simulink model "SUB_CanDm1"  (R2018b)
settings: Solver=VariableStepDiscrete  StartTime=0.0  StopTime=10  RelTol=1e-3
PreLoadFcn:
  | if(exist('MBDS_ModelCallback', 'file'))
  |    MBDS_ModelCallback('PreLoad');
  | end
PostLoadFcn:
  | if(exist('MBDS_ModelCallback', 'file'))
  |    MBDS_ModelCallback('PostLoad');
  | end
InitFcn:
  | if(exist('MBDS_ModelCallback', 'file'))
  |    MBDS_ModelCallback('Init');
  | end
StartFcn:
  | if(exist('MBDS_ModelCallback', 'file'))
  |    MBDS_ModelCallback('Start');
  | end
StopFcn:
  | if(exist('MBDS_ModelCallback', 'file'))
  |    MBDS_ModelCallback('Stop');
  | end
undefined symbols (not defined in the file): sigbuilder_block
libraries: KIBES_Signal x47, simulink x1
(part 1 of 2)
PreSaveFcn:
  | if(exist('MBDS_ModelCallback', 'file'))
  |    MBDS_ModelCallback('PreSave');
  | end
CloseFcn:
  | if(exist('MBDS_ModelCallback', 'file'))
  |    MBDS_ModelCallback('Close');
  | end
Description:
  | Design model of an MBDS Subsystem
settings Model: IsTargetCode=false  MBDS_Version=08.20  Creator=Marcio Kopke (uid96494)  LastModifiedBy=uid96494
settings ConfigSet: Description=MBDS configuration set optimized for simulation of model designs for automotive embedded systems.
settings SolverCC: MinimalZcImpactIntegration=on
settings DataIOCC: MaxDataPoints=100  SaveFormat=StructureWithTime  SaveOutput=off  DSMLogging=off  VisualizeSimOutput=off  SaveTime=off  SignalLoggingName=LogSignals
settings OptimizationCC: UseDivisionForNetSlopeComputation=UseDivisionForReciprocalsOfIntegersOnly  UseFloatMulNetSlope=on  DefaultUnderspecifiedDataType=single  OptimizeBlockIOStorage=off  BufferReuse=off  GlobalBufferReuse=off  StrengthReduction=on  ExpressionFolding=off  ExpressionDepthLimit=2147483647  LocalBlockOutputs=off  EfficientFloat2IntCast=on  LifeSpan=inf  BufferReusableBoundary=off  OptimizeBlockOrder=speed  OptimizeDataStoreBuffers=off  BusAssignmentInplaceUpdate=off  LabelGuidedReuse=on
settings DebuggingCC: SignalInfNanChecking=error  AlgebraicLoopMsg=error  ArtificialAlgebraicLoopMsg=error  UnderspecifiedInitializationDetection=Classic  CheckExecutionContextPreStartOutputMsg=on  CheckExecutionContextRuntimeOutputMsg=on  BlockPriorityViolationMsg=error  MinStepSizeMsg=error  TimeAdjustmentMsg=warning  SolverPrmCheckMsg=error  InheritedTsInSrcMsg=none  SingleTaskRateTransMsg=error  TasksWithSamePriorityMsg=error  SigSpecEnsureSampleTimeMsg=error  CheckMatrixSingularityMsg=error  ParameterUnderflowMsg=error  ParameterTunabilityLossMsg=error  FixptConstUnderflowMsg=warning  FixptConstOverflowMsg=warning  FixptConstPrecisionLossMsg=warning  VectorMatrixConversionMsg=error  SignalLabelMismatchMsg=warning  SFcnCompatibilityMsg=error  FrameProcessingCompatibilityMsg=warning  UniqueDataStoreMsg=error  BusObjectLabelMismatch=error  RootOutportRequireBusObject=error  AllowSymbolicDim=off  ModelReferenceIOMsg=error  ModelReferenceIOMismatchMessage=error  UnknownTsInhSupMsg=error  ModelReferenceDataLoggingMessage=error  StateNameClashWarn=warning  SimStateOlderReleaseMsg=warning  StrictBusMsg=ErrorOnBusTreatedAsVector  NonBusSignalsTreatedAsBus=error  SFInvalidInputDataAccessInChartInitDiag=error  SFTransitionOutsideNaturalParentDiag=error  SFUnreachableExecutionPathDiag=error  SFUndirectedBroadcastEventsDiag=error  SFTransitionActionBeforeConditionDiag=error  SFTemporalDelaySmallerThanSampleTimeDiag=error  SFExecutionAtInitializationDiag=none
settings HardwareCC: ProdBitPerPointer=32  ProdBitPerSizeT=32  ProdBitPerPtrDiffT=32  ProdLargestAtomicInteger=Long  ProdEndianess=BigEndian  ProdWordSize=32  ProdLongLongMode=on  ProdHWDeviceType=Custom Processor  TargetHWDeviceType=32-bit Generic
settings ModelReferenceCC: PropagateSignalLabelsOutOfModel=off
settings SFSimCC: SimUseLocalCustomCode=off  SimGenImportedTypeDefs=on  CompileTimeRecursionLimit=0  EnableRuntimeRecursion=off  MATLABDynamicMemAlloc=off  DefaultCustomCodeFunctionArrayLayout=Column-major
settings RTWCC: SystemTargetFile=MBDS.tlc  GenCodeOnly=on  TemplateMakefile=MBDS.tmf  Description=MBDS Target  GenerateReport=on  RTWUseLocalCustomCode=off  IncludeHyperlinkInReport=on  LaunchReport=on  GenerateTraceReport=on  GenerateTraceReportSl=on  GenerateTraceReportSf=on  GenerateTraceReportEml=on  GenerateCodeMetricsReport=on  RTWCompilerOptimization=on
settings CodeAppCC: ForceParamTrailComments=on  IgnoreCustomStorageClasses=off  OperatorAnnotations=on  SimulinkDataObjDesc=on  SFDataObjDesc=on  MangleLength=2  CustomSymbolStrType=$N$R$M  CustomSymbolStrFcn=$R$M  CustomSymbolStrUtil=$n$C  InsertBlockDesc=on  StateflowObjectComments=on  MATLABSourceComments=on  ReqsInCode=on  UseSimReservedNames=on
settings STFCustomTargetCC: UtilityFuncGeneration=Shared location  MultiwordLength=256  DynamicStringBufferSize=2  InferredTypesCompatibility=on  ModelReferenceCompliant=off  IncludeMdlTerminateFcn=off  CombineOutputUpdateFcns=on  CombineSignalStateStructs=on  SuppressErrorStatus=on  ERTCustomFileBanners=on  SupportComplex=off  SupportContinuousTime=off  SupportNonInlinedSFcns=off  RemoveDisableFunc=on  RemoveResetFunc=on  ParenthesesLevel=Maximum  CastingMode=Standards  MATLABClassNameForMDSCustomization=Simulink.SoftwareTarget.ERTCustomization  GenerateSharedConstants=off  SystemTargetFile=MBDS.tlc
settings ERTTargetCC: UtilityFuncGeneration=Shared location  DynamicStringBufferSize=2  InferredTypesCompatibility=on  ModelReferenceCompliant=off  ParMdlRefBuildCompliant=off  CompOptLevelCompliant=off  ConcurrentExecutionCompliant=off  IncludeMdlTerminateFcn=off  CombineSignalStateStructs=on  SuppressErrorStatus=on  SupportComplex=off  RemoveDisableFunc=on  ParenthesesLevel=Maximum  CastingMode=Standards  ModelStepFunctionPrototypeControlCompliant=off  CPPClassGenCompliant=off  UseToolchainInfoCompliant=off  GenerateSharedConstants=off  ERTCustomFileTemplate=example_file_process.tlc  EnableDataOwnership=on  PreserveExpressionOrder=on  PreserveIfCondition=on  SuppressUnreachableDefaultCases=off  EnableSignedLeftShifts=off  EnableSignedRightShifts=off  IndentStyle=Allman  NewlineStyle=CR+LF
settings ConfigComp: CovScope=ReferencedModels  CovIncludeTopModel=off  CovPath=SUB_CanDm1/Model/SUB_CanDm1_  CovSaveName=covData  CovMetricSettings=dsw  CovFilter=MBDS_CoverageFilter  CovHTMLOptions=-sRT=1 -sVT=0 -aTS=1 -bRG=1 -bTC=1 -hTR=1 -nFC=0 -nFD=0 -scm=1 -bcm=1 -xEv=0 -xEM=1  CovHtmlReporting=on  CovSaveOutputData=off  CovDataFileName=covData  CovShowResultsExplorer=off  CovExternalEMLEnable=off  CovSFcnEnable=off

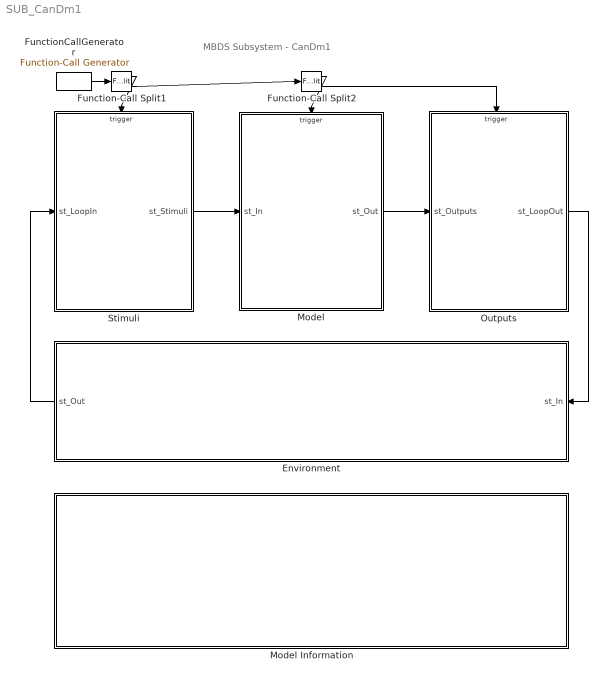
== system SUB_CanDm1 ==
  note: MBDS Subsystem - CanDm1
  Environment : Subsystem  Description=Environment subsystem for a MBDS model.
  Function-Call Split1 : FunctionCallSplit  InitFcn=|  NumOutputPorts=2
      | try
      |    MBDS_BlockCallback('Update', gcb);
      | end
      | try
      |    MBDS_BlockCallback('Update', gcb);
      | end
  Function-Call Split2 : FunctionCallSplit  InitFcn=|  NumOutputPorts=2
      | try
      |    MBDS_BlockCallback('Update', gcb);
      | end
      | try
      |    MBDS_BlockCallback('Update', gcb);
      | end
  FunctionCallGenerator : simulink/Ports & Subsystems/Function-Call Generator  sample_time=0.01  numberOfIterations=1
      settings: AttributesFormatString=Ts = %<sample_time>
  Model : Subsystem  Description=Model subsystem for a MBDS model. Here, the input signals to the model functionality are resolved from the Stimuli bus and the output signals of the model functionality are summarized into the Results bus.
  Model Information : Subsystem  InitFcn=|  mask(ModelInformation){MBDS_LibraryBlock=on, Company=-, Department=-, Responsible=-, Status=In Work, Complete=on, Check=on, Test=on, Optimize=on, Documentation=on, FcnErrors=off, GenericToDo=off, DocumentState=Draft, GenericToDoName=Enter a user specific ToDo text, MBDS_BlockVersion=07.00}
      | if(exist('MBDS_BlockCallback', 'file'))
      |    MBDS_BlockCallback('Update', gcb);
      | end
      mask prompts: MBDS_LibraryBlock "MBDS Library Block"; Complete "Complete Implementation"; Check "Check Modelling Guidelines"; Test "Test Functionality"; Optimize "Optimize Implementation"; Documentation "Create Documentation"; FcnErrors "Remove Functional Errors"; GenericToDo "Enter a user specific ToDo text"; DocumentState "Document State:"; GenericToDoName "Generic ToDo Name:"; MBDS_BlockVersion "Block version:"
      mask help: This block displays model information and ToDo's on it's block mask. Via the block parameter mask further model information and configuration options can be accessed.
      mask init:
      | if(exist('MBDS_BlockCallback', 'file'))
      |    MBDS_BlockCallback('Copy', gcb);    
      | end
      mask Help: eval(['open([workdir(''library_dir:''),''\Blockset\help\'',get_param(gcb,''MaskType''),''.html''])'])
      mask TypeOptions Status: In Work | Done
      mask TypeOptions DocumentState: Draft | Final | Released
      mask Callback GenericToDoName:
      | MaskPrompts = get_param(gcb, 'MaskPrompts');
      | MaskPrompts{12} = get_param(gcb, 'GenericToDoName');
      | if(length(MaskPrompts{12}) > 75)
      |    MaskPrompts{12} = MaskPrompts{12}(1:75);
      |    set_param(gcb, 'GenericToDoName', MaskPrompts{12});
      | end
      | set_param(gcb, 'MaskPrompts', MaskPrompts);
      | clear MaskPrompts;
      mask DialogControl ParameterTabVar0 Prompt: Info
      mask DialogControl ParameterTabVar01 Prompt: ToDo's
      mask DialogControl ParameterTabVar012 Prompt: Options
      mask DialogControl ParameterTabVar0123 Prompt: Version
      mask Display:
      | % Get ToDo's
      | IsComplete       = strcmpi(Complete, 'on');
      | IsOptimize       = strcmpi(Optimize, 'on');
      | IsCheck          = strcmpi(Check, 'on');
      | IsDocumentation  = strcmpi(Documentation, 'on');
      | IsTest           = strcmpi(Test, 'on');
      | IsFcnErrors      = strcmpi(FcnErrors, 'on');
      | IsGenericToDo    = strcmpi(GenericToDo, 'on');
      | 
      | % Determine status
      | if(IsFcnErrors || IsTest || IsComplete || IsDocumentation || IsCheck || IsOptimize || IsGenericToDo)
      |    Status = 'In Work';
      | else
      |    Status = 'Done';
      | end
      | 
      | % Update status parameter
      | if(~strcmpi(get_param(gcb, 'Status'), Status))
      |    set_param(gcb, 'Status', Status);
      | end
      | 
      | % Determine severity
      | if(IsFcnErrors)
      |    % Severity: Critical
      |    BoxColorFile = 'Box_Red.tif';
      |    IconFile     = 'State_Red.jpg';
      | elseif (IsTest || IsComplete || IsGenericToDo)
      |    % Severity: Major
      |    BoxColorFile = 'Box_Orange.tif';
      |    IconFile     = 'State_Orange.jpg';
      | elseif (IsDocumentation || IsCheck || IsOptimize)
      |    % Severity: Minor
      |    BoxColorFile = 'Box_Grey.tif';
      |    IconFile     = 'State_Grey.jpg';
      | else
      |    % Severity: None
      |    BoxColorFile = 'Box_Green.tif';
      |    IconFile     = 'State_Green.jpg';
      | end
      | 
      | % Display Model Information
      | InfoStr1 = sprintf('%s', get_param(bdroot, 'Name'));
      | InfoStr2 = sprintf('Model Version:  %s', get_param(bdroot, 'ModelVersion'));
      | InfoStr3 = sprintf('Company:  %s', Company);
      | InfoStr4 = sprintf('Department:  %s', Department);
      | InfoStr5 = sprintf('Responsible:  %s', Responsible);
      | InfoStr6 = sprintf('Last Modified by:  %s at %s', get_param(bdroot, 'LastModifiedBy'), get_param(bdroot, 'LastModifiedDate'));
      | %Y is to do!!!!
      | text(0.5, 0.69, sprintf('%s\n%s\n%s\n%s\n%s\n%s\n%s', InfoStr1, InfoStr2, InfoStr3, InfoStr4, InfoStr5, InfoStr6), 'horizontalAlignment', 'center');
      | clear InfoStr1 InfoStr2 InfoStr3 InfoStr4 InfoStr5 InfoStr6;
      | 
      | % Display Status
      | if(exist(BoxColorFile, 'file'))
      |    image(imread(BoxColorFile,'tif'), [0,0,1,0.45]);
      | end
      | if(exist(IconFile, 'file'))
      |    image(imread(IconFile,'jpg'), [0.025,0.09,0.08,0.26]);
      |    image(imread(IconFile,'jpg'), [0.9,0.09,0.08,0.26]);
      | end
      | plot([-0.01 1.01], [0.45 0.45])
      | text(0.5, 0.38, sprintf('Status: %s', upper(Status)), 'horizontalAlignment', 'center');
      | 
      | % Display ToDo's
      | if(IsComplete)
      |    text(0.15, 0.31, '- Complete Implementation');
      | end
      | if(IsOptimize)
      |    text(0.6, 0.31, '- Optimize Implementation');
      | end
      | 
      | if(IsCheck)
      |    text(0.15, 0.23, '- Check Modeling Guidelines');
      | end
      | if(IsDocumentation)
      |    text(0.6, 0.23, '- Create Documentation');
      | end
      | 
      | if(IsTest)
      |    text(0.15, 0.14, '- Test Functionality');
      | end
      | if(IsFcnErrors)
      |    text(0.6, 0.14, '- Remove Functional Errors');
      | end
      | 
      | if(IsGenericToDo)
      |    text(0.15, 0.06, ['- ', GenericToDoName]);
      | end
  Outputs : Subsystem  Description=Result subsystem for a MBDS model. Here, output signals from the model functionality can be displayed using a scope or display. Additionally, the output signals can be postprocessed before they will passed to the feedback loop.
  Stimuli : Subsystem  Description=Stimuli subsystem for a MBDS model. Here, input signals for testing the model functionality can be defined using the signal builder or calculated applying arbitrary basic-blocks. Additionally, feedback signals can be preprocessed at this stage.
  wires:
  Model/1(st_Out) -> Outputs/1(st_Outputs)
  Stimuli/1(st_Stimuli) -> Model/1(st_In)
  Outputs/1(st_LoopOut) -> Environment/1(st_In)
  Environment/1(st_Out) -> Stimuli/1(st_LoopIn)
  FunctionCallGenerator/1 -> Function-Call Split1/1
  Function-Call Split1/2 -> Function-Call Split2/1
  Function-Call Split1/1 -> Stimuli/Trigger
  Function-Call Split2/1 -> Model/Trigger
  Function-Call Split2/2 -> Outputs/Trigger

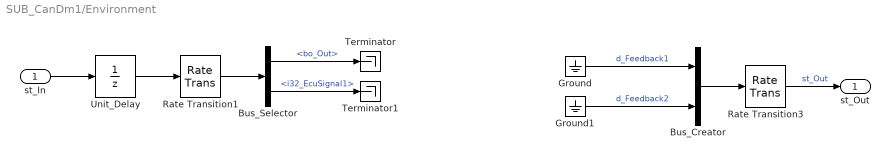
== system SUB_CanDm1/Environment ==
  st_In : Inport
  Bus_Creator : BusCreator  InitFcn=|  Inputs=2
      | try
      |    MBDS_BlockCallback('Update', gcb);
      | end
      | try
      |    MBDS_BlockCallback('Update', gcb);
      | end
  Bus_Selector : BusSelector  InitFcn=|  OutputSignals=st_Outputs.bo_Out,i32_EcuSignal1
      | try
      |    MBDS_BlockCallback('Update', gcb);
      | end
      | try
      |    MBDS_BlockCallback('Update', gcb);
      | end
  Ground : Ground  InitFcn=|
      | try
      |    MBDS_BlockCallback('Update', gcb);
      | end
  Ground1 : Ground  InitFcn=|
      | try
      |    MBDS_BlockCallback('Update', gcb);
      | end
  Rate Transition1 : RateTransition  InitFcn=|  OutPortSampleTimeOpt=Inherit
      | try
      |    MBDS_BlockCallback('Update', gcb);
      | end
  Rate Transition3 : RateTransition  InitFcn=|  OutPortSampleTimeOpt=Inherit
      | try
      |    MBDS_BlockCallback('Update', gcb);
      | end
  Terminator : Terminator
      settings: MoveFcn=UpdateBlockSize(gcb);
      settings: InitFcn=|
      | try
      |    MBDS_BlockCallback('Update', gcb);
      | end
  Terminator1 : Terminator
      settings: MoveFcn=UpdateBlockSize(gcb);
      settings: InitFcn=|
      | try
      |    MBDS_BlockCallback('Update', gcb);
      | end
  Unit_Delay : UnitDelay  InitFcn=|  SampleTime=-1
      | try
      |    MBDS_BlockCallback('Update', gcb);
      | end
      | try                                  
      |    MBDS_BlockCallback('Update', gcb);
      | end
      settings: AttributesFormatString=Init = %<X0>
  st_Out : Outport
  wires:
  Bus_Creator/1 -> Rate Transition3/1
  st_In/1 -> Unit_Delay/1
  Ground/1 -> Bus_Creator/1  "d_Feedback1"
  Ground1/1 -> Bus_Creator/2  "d_Feedback2"
  Unit_Delay/1 -> Rate Transition1/1
  Rate Transition3/1 -> st_Out/1  "st_Out"
  Rate Transition1/1 -> Bus_Selector/1
  Bus_Selector/1 -> Terminator/1  "<bo_Out>"
  Bus_Selector/2 -> Terminator1/1  "<i32_EcuSignal1>"

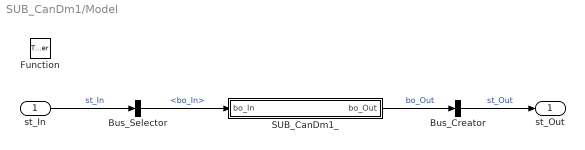
== system SUB_CanDm1/Model ==
  st_In : Inport
      settings: LatchInputForFeedbackSignals=on
  Function : TriggerPort  InitFcn=|  TriggerType=function-call  VariantControl=(inherit)
      | try
      |    MBDS_BlockCallback('Update', gcb);
      | end
  Bus_Creator : BusCreator  InitFcn=|  Inputs=1
      | try
      |    MBDS_BlockCallback('Update', gcb);
      | end
      | try
      |    MBDS_BlockCallback('Update', gcb);
      | end
  Bus_Selector : BusSelector  InitFcn=|  OutputSignals=bo_In
      | try
      |    MBDS_BlockCallback('Update', gcb);
      | end
      | try
      |    MBDS_BlockCallback('Update', gcb);
      | end
  SUB_CanDm1_ : Subsystem  Tag=Functionality  Description=Check DM1 Rx/Tx
      settings: AttributesFormatString=Functionality
  st_Out : Outport
  wires:
  st_In/1 -> Bus_Selector/1  "st_In"
  Bus_Creator/1 -> st_Out/1  "st_Out"
  Bus_Selector/1 -> SUB_CanDm1_/1(bo_In)  "<bo_In>"
  SUB_CanDm1_/1(bo_Out) -> Bus_Creator/1  "bo_Out"

== system SUB_CanDm1/Model Information ==
  note: Double Click the Model Information block to open the block parameter mask

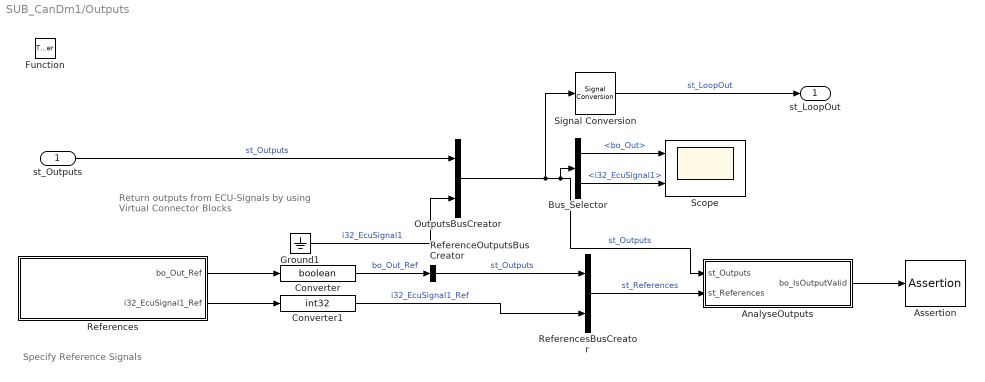
== system SUB_CanDm1/Outputs ==
  note: Specify Reference Signals
  note: Return outputs from ECU-Signals
      | by using Virtual Connector Blocks
  st_Outputs : Inport
      settings: LatchInputForFeedbackSignals=on
  Function : TriggerPort  InitFcn=|  TriggerType=function-call  VariantControl=(inherit)
      | try
      |    MBDS_BlockCallback('Update', gcb);
      | end
  AnalyseOutputs : Subsystem
  Assertion : Assertion  Enabled=off
  Bus_Selector : BusSelector  InitFcn=|  OutputSignals=st_Outputs.bo_Out,i32_EcuSignal1
      | try
      |    MBDS_BlockCallback('Update', gcb);
      | end
      | try
      |    MBDS_BlockCallback('Update', gcb);
      | end
  Converter : DataTypeConversion  InitFcn=|  OutDataTypeStr=boolean  SaturateOnIntegerOverflow=on
      | try
      |    MBDS_BlockCallback('Update', gcb);
      | end
      settings: AttributesFormatString=Saturate: %<SaturateOnIntegerOverflow>
  Converter1 : DataTypeConversion  InitFcn=|  OutDataTypeStr=int32  SaturateOnIntegerOverflow=on
      | try
      |    MBDS_BlockCallback('Update', gcb);
      | end
      settings: AttributesFormatString=Saturate: %<SaturateOnIntegerOverflow>
  Ground1 : Ground  InitFcn=|
      | try
      |    MBDS_BlockCallback('Update', gcb);
      | end
      | try
      |    MBDS_BlockCallback('Update', gcb);
      | end
  OutputsBusCreator : BusCreator  InitFcn=|  Inputs=2
      | try
      |    MBDS_BlockCallback('Update', gcb);
      | end
      | try
      |    MBDS_BlockCallback('Update', gcb);
      | end
  ReferenceOutputsBusCreator : BusCreator  InitFcn=|  Inputs=1
      | try
      |    MBDS_BlockCallback('Update', gcb);
      | end
      | try
      |    MBDS_BlockCallback('Update', gcb);
      | end
  References : Subsystem  Tag=STV Subsys  LoadFcn=sigbuilder_block('load');  StartFcn=sigbuilder_block('start');  StopFcn=sigbuilder_block('stop');  ClipboardFcn=sigbuilder_block('clipboard');  mask(Sigbuilder block){tuvar=[0:10]}
      mask init:
      | if ~strcmp(get_param(bdroot(gcb),'SimulationStatus'),'stopped'),tuvar = sigbuilder_block('maskInit'); end
      settings: CopyFcn=sigbuilder_block('copy');  DeleteFcn=sigbuilder_block('delete');  ModelCloseFcn=sigbuilder_block('modelClose');  PreSaveFcn=sigbuilder_block('preSave');  PauseFcn=sigbuilder_block('pause');  ContinueFcn=sigbuilder_block('continue');  NameChangeFcn=sigbuilder_block('namechange');  OpenFcn=sigbuilder_block('open',[50 50 520 400 ]);  CloseFcn=sigbuilder_block('close');
      mask Display: plot(0, 0, 100, 100,[2, 2, 32, 32, 2], [68, 8, 8, 68, 68],[32, 2], [38, 38], [32, 19, 2],[53, 60, 44], [32, 17, 17, 2],[16, 16, 31, 31]);txt = getActiveGroup(gcbh);text(2, 100, txt,'verticalAlignment', 'top');
  ReferencesBusCreator : BusCreator  InitFcn=|  Inputs=2
      | try
      |    MBDS_BlockCallback('Update', gcb);
      | end
      | try
      |    MBDS_BlockCallback('Update', gcb);
      | end
  Scope : Scope  NumInputPorts=2
  Signal Conversion : SignalConversion  InitFcn=|  OverrideOpt=off
      | try
      |    MBDS_BlockCallback('Update', gcb);
      | end
  st_LoopOut : Outport
  wires:
  AnalyseOutputs/1(bo_IsOutputValid) -> Assertion/1
  ReferencesBusCreator/1 -> AnalyseOutputs/2(st_References)  "st_References"
  st_Outputs/1 -> OutputsBusCreator/1  "st_Outputs"
  Ground1/1 -> OutputsBusCreator/2  "i32_EcuSignal1"
  OutputsBusCreator/1 -> AnalyseOutputs/1(st_Outputs), Bus_Selector/1, Signal Conversion/1  "st_Outputs"
  Signal Conversion/1 -> st_LoopOut/1  "st_LoopOut"
  Bus_Selector/1 -> Scope/1  "<bo_Out>"
  Bus_Selector/2 -> Scope/2  "<i32_EcuSignal1>"
  ReferenceOutputsBusCreator/1 -> ReferencesBusCreator/1  "st_Outputs"
  Converter/1 -> ReferenceOutputsBusCreator/1  "bo_Out_Ref"
  References/1(bo_Out_Ref) -> Converter/1
  References/2(i32_EcuSignal1_Ref) -> Converter1/1
  Converter1/1 -> ReferencesBusCreator/2  "i32_EcuSignal1_Ref"

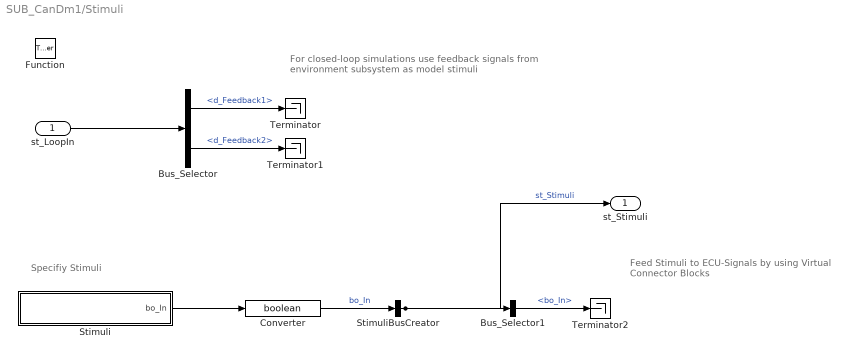
== system SUB_CanDm1/Stimuli ==
  note: Specifiy Stimuli
  note: For closed-loop simulations use feedback signals
      | from environment subsystem as model stimuli
  note: Feed Stimuli to ECU-Signals
      | by using Virtual Connector Blocks
  st_LoopIn : Inport
      settings: LatchInputForFeedbackSignals=on
  Function : TriggerPort  InitFcn=|  TriggerType=function-call  VariantControl=(inherit)
      | try
      |    MBDS_BlockCallback('Update', gcb);
      | end
  Bus_Selector : BusSelector  InitFcn=|  OutputSignals=d_Feedback1,d_Feedback2
      | try
      |    MBDS_BlockCallback('Update', gcb);
      | end
      | try
      |    MBDS_BlockCallback('Update', gcb);
      | end
  Bus_Selector1 : BusSelector  InitFcn=|  OutputSignals=bo_In
      | try
      |    MBDS_BlockCallback('Update', gcb);
      | end
      | try
      |    MBDS_BlockCallback('Update', gcb);
      | end
  Converter : DataTypeConversion  InitFcn=|  OutDataTypeStr=boolean  SaturateOnIntegerOverflow=on
      | try
      |    MBDS_BlockCallback('Update', gcb);
      | end
      settings: AttributesFormatString=Saturate: %<SaturateOnIntegerOverflow>
  Stimuli : Subsystem  Tag=STV Subsys  LoadFcn=sigbuilder_block('load');  StartFcn=sigbuilder_block('start');  StopFcn=sigbuilder_block('stop');  ClipboardFcn=sigbuilder_block('clipboard');  mask(Sigbuilder block){tuvar=[0:10]}
      mask init:
      | if ~strcmp(get_param(bdroot(gcb),'SimulationStatus'),'stopped'),tuvar = sigbuilder_block('maskInit'); end
      settings: CopyFcn=sigbuilder_block('copy');  DeleteFcn=sigbuilder_block('delete');  ModelCloseFcn=sigbuilder_block('modelClose');  PreSaveFcn=sigbuilder_block('preSave');  PauseFcn=sigbuilder_block('pause');  ContinueFcn=sigbuilder_block('continue');  NameChangeFcn=sigbuilder_block('namechange');  OpenFcn=sigbuilder_block('open',[50 50 520 400 ]);  CloseFcn=sigbuilder_block('close');
      mask Display: plot(0, 0, 100, 100,[2, 2, 32, 32, 2], [68, 8, 8, 68, 68],[32, 2], [38, 38], [32, 19, 2],[53, 60, 44], [32, 17, 17, 2],[16, 16, 31, 31]);txt = getActiveGroup(gcbh);text(2, 100, txt,'verticalAlignment', 'top');
  StimuliBusCreator : BusCreator  InitFcn=|  Inputs=1
      | try
      |    MBDS_BlockCallback('Update', gcb);
      | end
      | try
      |    MBDS_BlockCallback('Update', gcb);
      | end
  Terminator : Terminator
      settings: InitFcn=|
      | try
      |    MBDS_BlockCallback('Update', gcb);
      | end
      | try
      |    MBDS_BlockCallback('Update', gcb);
      | end
  Terminator1 : Terminator
      settings: InitFcn=|
      | try
      |    MBDS_BlockCallback('Update', gcb);
      | end
      | try
      |    MBDS_BlockCallback('Update', gcb);
      | end
  Terminator2 : Terminator
      settings: MoveFcn=UpdateBlockSize(gcb);
      settings: InitFcn=|
      | try
      |    MBDS_BlockCallback('Update', gcb);
      | end
  st_Stimuli : Outport
  wires:
  Bus_Selector/1 -> Terminator/1  "<d_Feedback1>"
  Bus_Selector/2 -> Terminator1/1  "<d_Feedback2>"
  st_LoopIn/1 -> Bus_Selector/1
  Bus_Selector1/1 -> Terminator2/1  "<bo_In>"
  StimuliBusCreator/1 -> st_Stimuli/1, Bus_Selector1/1  "st_Stimuli"
  Converter/1 -> StimuliBusCreator/1  "bo_In"
  Stimuli/1(bo_In) -> Converter/1

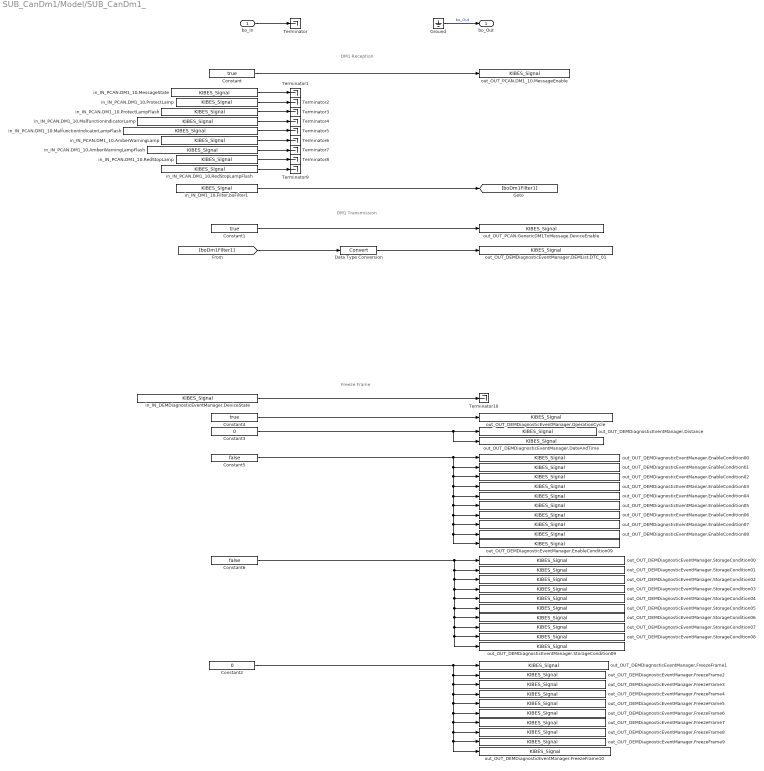
== system SUB_CanDm1/Model/SUB_CanDm1_ ==
  note: DM1 Reception
  note: DM1 Transmission
  note: Freeze Frame
  bo_In : Inport  OutDataTypeStr=boolean
  Constant : Constant  InitFcn=|  Value=true  OutDataTypeStr=boolean
      | if(exist('MBDS_BlockCallback', 'file'))
      |    MBDS_BlockCallback('Update', gcb);  
      | end
  Constant1 : Constant  InitFcn=|  Value=true  OutDataTypeStr=boolean
      | if(exist('MBDS_BlockCallback', 'file'))
      |    MBDS_BlockCallback('Update', gcb);  
      | end
  Constant2 : Constant  InitFcn=|  Value=0  OutDataTypeStr=uint16
      | if(exist('MBDS_BlockCallback', 'file'))
      |    MBDS_BlockCallback('Update', gcb);  
      | end
  Constant3 : Constant  InitFcn=|  Value=0  OutDataTypeStr=uint32
      | if(exist('MBDS_BlockCallback', 'file'))
      |    MBDS_BlockCallback('Update', gcb);  
      | end
  Constant4 : Constant  InitFcn=|  Value=true  OutDataTypeStr=boolean
      | if(exist('MBDS_BlockCallback', 'file'))
      |    MBDS_BlockCallback('Update', gcb);  
      | end
  Constant5 : Constant  InitFcn=|  Value=false  OutDataTypeStr=boolean
      | if(exist('MBDS_BlockCallback', 'file'))
      |    MBDS_BlockCallback('Update', gcb);  
      | end
  Constant6 : Constant  InitFcn=|  Value=false  OutDataTypeStr=boolean
      | if(exist('MBDS_BlockCallback', 'file'))
      |    MBDS_BlockCallback('Update', gcb);  
      | end
  Data Type Conversion : DataTypeConversion  InitFcn=|
      | try
      |    MBDS_BlockCallback('Update', gcb);
      | end
      settings: AttributesFormatString=Saturate: %<SaturateOnIntegerOverflow>
  Ground : Ground  InitFcn=|
      | try
      |    MBDS_BlockCallback('Update', gcb);
      | end
      settings: MoveFcn=UpdateBlockSize(gcb);
  Terminator{,1..10} (11 alike) : Terminator
      settings: MoveFcn=UpdateBlockSize(gcb);
      settings: InitFcn=|
      | try
      |    MBDS_BlockCallback('Update', gcb);
      | end
  in_IN_DEMDiagnosticEventManager.DeviceState : KIBES_Signal/KIBES_Signal  MBDS_LibraryBlock=on  DatabaseKey=2238  SignalName=IN_DEMDiagnosticEventManager.DeviceState  SymbolName=IN_DEMDiagnosticEventManager_DeviceState_002238  DataType=uint16  Init=0  Slope=1  Bias=0  DataSize=1  fpDataType=uint16  BlockIOType=Inport  DeviceType=0
  in_IN_DM1_10.Filter.boFilter1 : KIBES_Signal/KIBES_Signal  MBDS_LibraryBlock=on  DatabaseKey=2234  SignalName=IN_DM1_10.Filter.boFilter1  SymbolName=IN_DM1_10_Filter_boFilter1_002234  DataType=boolean  Init=0  Slope=1  Bias=0  DataSize=1  fpDataType=boolean  BlockIOType=Inport  DeviceType=0
  in_IN_PCAN.DM1_10.AmberWarningLamp : KIBES_Signal/KIBES_Signal  MBDS_LibraryBlock=on  DatabaseKey=2233  SignalName=IN_PCAN.DM1_10.AmberWarningLamp  SymbolName=IN_PCAN_DM1_10_AmberWarningLamp_002233  DataType=boolean  Init=0  Slope=1  Bias=0  DataSize=1  fpDataType=boolean  BlockIOType=Inport  DeviceType=0
  in_IN_PCAN.DM1_10.AmberWarningLampFlash : KIBES_Signal/KIBES_Signal  MBDS_LibraryBlock=on  DatabaseKey=2232  SignalName=IN_PCAN.DM1_10.AmberWarningLampFlash  SymbolName=IN_PCAN_DM1_10_AmberWarningLampFlash_002232  DataType=uint8  Init=0  Slope=1  Bias=0  DataSize=1  fpDataType=uint8  BlockIOType=Inport  DeviceType=0
  in_IN_PCAN.DM1_10.MalfunctionIndicatorLamp : KIBES_Signal/KIBES_Signal  MBDS_LibraryBlock=on  DatabaseKey=2231  SignalName=IN_PCAN.DM1_10.MalfunctionIndicatorLamp  SymbolName=IN_PCAN_DM1_10_MalfunctionIndicatorLamp_002231  DataType=boolean  Init=0  Slope=1  Bias=0  DataSize=1  fpDataType=boolean  BlockIOType=Inport  DeviceType=0
  in_IN_PCAN.DM1_10.MalfunctionIndicatorLampFlash : KIBES_Signal/KIBES_Signal  MBDS_LibraryBlock=on  DatabaseKey=2230  SignalName=IN_PCAN.DM1_10.MalfunctionIndicatorLampFlash  SymbolName=IN_PCAN_DM1_10_MalfunctionIndicatorLampFlash_002230  DataType=uint8  Init=0  Slope=1  Bias=0  DataSize=1  fpDataType=uint8  BlockIOType=Inport  DeviceType=0
  in_IN_PCAN.DM1_10.MessageState : KIBES_Signal/KIBES_Signal  MBDS_LibraryBlock=on  DatabaseKey=2228  SignalName=IN_PCAN.DM1_10.MessageState  SymbolName=IN_PCAN_DM1_10_MessageState_002228  DataType=uint16  Init=0  Slope=1  Bias=0  DataSize=1  fpDataType=uint16  BlockIOType=Inport  DeviceType=0
  in_IN_PCAN.DM1_10.ProtectLamp : KIBES_Signal/KIBES_Signal  MBDS_LibraryBlock=on  DatabaseKey=2227  SignalName=IN_PCAN.DM1_10.ProtectLamp  SymbolName=IN_PCAN_DM1_10_ProtectLamp_002227  DataType=boolean  Init=0  Slope=1  Bias=0  DataSize=1  fpDataType=boolean  BlockIOType=Inport  DeviceType=0
  in_IN_PCAN.DM1_10.ProtectLampFlash : KIBES_Signal/KIBES_Signal  MBDS_LibraryBlock=on  DatabaseKey=2226  SignalName=IN_PCAN.DM1_10.ProtectLampFlash  SymbolName=IN_PCAN_DM1_10_ProtectLampFlash_002226  DataType=uint8  Init=0  Slope=1  Bias=0  DataSize=1  fpDataType=uint8  BlockIOType=Inport  DeviceType=0
  in_IN_PCAN.DM1_10.RedStopLamp : KIBES_Signal/KIBES_Signal  MBDS_LibraryBlock=on  DatabaseKey=2225  SignalName=IN_PCAN.DM1_10.RedStopLamp  SymbolName=IN_PCAN_DM1_10_RedStopLamp_002225  DataType=boolean  Init=0  Slope=1  Bias=0  DataSize=1  fpDataType=boolean  BlockIOType=Inport  DeviceType=0
  in_IN_PCAN.DM1_10.RedStopLampFlash : KIBES_Signal/KIBES_Signal  MBDS_LibraryBlock=on  DatabaseKey=2224  SignalName=IN_PCAN.DM1_10.RedStopLampFlash  SymbolName=IN_PCAN_DM1_10_RedStopLampFlash_002224  DataType=uint8  Init=0  Slope=1  Bias=0  DataSize=1  fpDataType=uint8  BlockIOType=Inport  DeviceType=0
  out_OUT_DEMDiagnosticEventManager.DEMList.DTC_01 : KIBES_Signal/KIBES_Signal  MBDS_LibraryBlock=on  DatabaseKey=2237  SignalName=OUT_DEMDiagnosticEventManager.DEMList.DTC_01  SymbolName=OUT_DEMDiagnosticEventManager_DEMList_DTC_01_002237  DataType=uint8  Init=0  Slope=1  Bias=0  DataSize=1  fpDataType=uint8  BlockIOType=Outport  DeviceType=0
  out_OUT_DEMDiagnosticEventManager.DateAndTime : KIBES_Signal/KIBES_Signal  MBDS_LibraryBlock=on  DatabaseKey=2242  SignalName=OUT_DEMDiagnosticEventManager.DateAndTime  SymbolName=OUT_DEMDiagnosticEventManager_DateAndTime_002242  DataType=uint32  Init=0  Slope=1  Bias=0  DataSize=1  fpDataType=uint32  BlockIOType=Outport  DeviceType=0
  out_OUT_DEMDiagnosticEventManager.Distance : KIBES_Signal/KIBES_Signal  MBDS_LibraryBlock=on  DatabaseKey=2243  SignalName=OUT_DEMDiagnosticEventManager.Distance  SymbolName=OUT_DEMDiagnosticEventManager_Distance_002243  DataType=uint32  Init=0  Slope=1  Bias=0  DataSize=1  fpDataType=uint32  BlockIOType=Outport  DeviceType=0
  out_OUT_DEMDiagnosticEventManager.EnableCondition00 : KIBES_Signal/KIBES_Signal  MBDS_LibraryBlock=on  DatabaseKey=2239  SignalName=OUT_DEMDiagnosticEventManager.EnableCondition00  SymbolName=OUT_DEMDiagnosticEventManager_EnableCondition00_002239  DataType=boolean  Init=0  Slope=1  Bias=0  DataSize=1  fpDataType=boolean  BlockIOType=Outport  DeviceType=0
  out_OUT_DEMDiagnosticEventManager.EnableCondition01 : KIBES_Signal/KIBES_Signal  MBDS_LibraryBlock=on  DatabaseKey=2245  SignalName=OUT_DEMDiagnosticEventManager.EnableCondition01  SymbolName=OUT_DEMDiagnosticEventManager_EnableCondition01_002245  DataType=boolean  Init=0  Slope=1  Bias=0  DataSize=1  fpDataType=boolean  BlockIOType=Outport  DeviceType=0
  out_OUT_DEMDiagnosticEventManager.EnableCondition02 : KIBES_Signal/KIBES_Signal  MBDS_LibraryBlock=on  DatabaseKey=2246  SignalName=OUT_DEMDiagnosticEventManager.EnableCondition02  SymbolName=OUT_DEMDiagnosticEventManager_EnableCondition02_002246  DataType=boolean  Init=0  Slope=1  Bias=0  DataSize=1  fpDataType=boolean  BlockIOType=Outport  DeviceType=0
  out_OUT_DEMDiagnosticEventManager.EnableCondition03 : KIBES_Signal/KIBES_Signal  MBDS_LibraryBlock=on  DatabaseKey=2247  SignalName=OUT_DEMDiagnosticEventManager.EnableCondition03  SymbolName=OUT_DEMDiagnosticEventManager_EnableCondition03_002247  DataType=boolean  Init=0  Slope=1  Bias=0  DataSize=1  fpDataType=boolean  BlockIOType=Outport  DeviceType=0
  out_OUT_DEMDiagnosticEventManager.EnableCondition04 : KIBES_Signal/KIBES_Signal  MBDS_LibraryBlock=on  DatabaseKey=2248  SignalName=OUT_DEMDiagnosticEventManager.EnableCondition04  SymbolName=OUT_DEMDiagnosticEventManager_EnableCondition04_002248  DataType=boolean  Init=0  Slope=1  Bias=0  DataSize=1  fpDataType=boolean  BlockIOType=Outport  DeviceType=0
  out_OUT_DEMDiagnosticEventManager.EnableCondition05 : KIBES_Signal/KIBES_Signal  MBDS_LibraryBlock=on  DatabaseKey=2249  SignalName=OUT_DEMDiagnosticEventManager.EnableCondition05  SymbolName=OUT_DEMDiagnosticEventManager_EnableCondition05_002249  DataType=boolean  Init=0  Slope=1  Bias=0  DataSize=1  fpDataType=boolean  BlockIOType=Outport  DeviceType=0
  out_OUT_DEMDiagnosticEventManager.EnableCondition06 : KIBES_Signal/KIBES_Signal  MBDS_LibraryBlock=on  DatabaseKey=2250  SignalName=OUT_DEMDiagnosticEventManager.EnableCondition06  SymbolName=OUT_DEMDiagnosticEventManager_EnableCondition06_002250  DataType=boolean  Init=0  Slope=1  Bias=0  DataSize=1  fpDataType=boolean  BlockIOType=Outport  DeviceType=0
  out_OUT_DEMDiagnosticEventManager.EnableCondition07 : KIBES_Signal/KIBES_Signal  MBDS_LibraryBlock=on  DatabaseKey=2251  SignalName=OUT_DEMDiagnosticEventManager.EnableCondition07  SymbolName=OUT_DEMDiagnosticEventManager_EnableCondition07_002251  DataType=boolean  Init=0  Slope=1  Bias=0  DataSize=1  fpDataType=boolean  BlockIOType=Outport  DeviceType=0
  out_OUT_DEMDiagnosticEventManager.EnableCondition08 : KIBES_Signal/KIBES_Signal  MBDS_LibraryBlock=on  DatabaseKey=2252  SignalName=OUT_DEMDiagnosticEventManager.EnableCondition08  SymbolName=OUT_DEMDiagnosticEventManager_EnableCondition08_002252  DataType=boolean  Init=0  Slope=1  Bias=0  DataSize=1  fpDataType=boolean  BlockIOType=Outport  DeviceType=0
  out_OUT_DEMDiagnosticEventManager.EnableCondition09 : KIBES_Signal/KIBES_Signal  MBDS_LibraryBlock=on  DatabaseKey=2244  SignalName=OUT_DEMDiagnosticEventManager.EnableCondition09  SymbolName=OUT_DEMDiagnosticEventManager_EnableCondition09_002244  DataType=boolean  Init=0  Slope=1  Bias=0  DataSize=1  fpDataType=boolean  BlockIOType=Outport  DeviceType=0
  out_OUT_DEMDiagnosticEventManager.FreezeFrame1 : KIBES_Signal/KIBES_Signal  MBDS_LibraryBlock=on  DatabaseKey=2241  SignalName=OUT_DEMDiagnosticEventManager.FreezeFrame1  SymbolName=OUT_DEMDiagnosticEventManager_FreezeFrame1_002241  DataType=uint16  Init=0  Slope=1  Bias=0  DataSize=1  fpDataType=uint16  BlockIOType=Outport  DeviceType=0
  out_OUT_DEMDiagnosticEventManager.FreezeFrame10 : KIBES_Signal/KIBES_Signal  MBDS_LibraryBlock=on  DatabaseKey=2270  SignalName=OUT_DEMDiagnosticEventManager.FreezeFrame10  SymbolName=OUT_DEMDiagnosticEventManager_FreezeFrame10_002270  DataType=uint16  Init=0  Slope=1  Bias=0  DataSize=1  fpDataType=uint16  BlockIOType=Outport  DeviceType=0
  out_OUT_DEMDiagnosticEventManager.FreezeFrame2 : KIBES_Signal/KIBES_Signal  MBDS_LibraryBlock=on  DatabaseKey=2253  SignalName=OUT_DEMDiagnosticEventManager.FreezeFrame2  SymbolName=OUT_DEMDiagnosticEventManager_FreezeFrame2_002253  DataType=uint16  Init=0  Slope=1  Bias=0  DataSize=1  fpDataType=uint16  BlockIOType=Outport  DeviceType=0
  out_OUT_DEMDiagnosticEventManager.FreezeFrame3 : KIBES_Signal/KIBES_Signal  MBDS_LibraryBlock=on  DatabaseKey=2254  SignalName=OUT_DEMDiagnosticEventManager.FreezeFrame3  SymbolName=OUT_DEMDiagnosticEventManager_FreezeFrame3_002254  DataType=uint16  Init=0  Slope=1  Bias=0  DataSize=1  fpDataType=uint16  BlockIOType=Outport  DeviceType=0
  out_OUT_DEMDiagnosticEventManager.FreezeFrame4 : KIBES_Signal/KIBES_Signal  MBDS_LibraryBlock=on  DatabaseKey=2255  SignalName=OUT_DEMDiagnosticEventManager.FreezeFrame4  SymbolName=OUT_DEMDiagnosticEventManager_FreezeFrame4_002255  DataType=uint16  Init=0  Slope=1  Bias=0  DataSize=1  fpDataType=uint16  BlockIOType=Outport  DeviceType=0
  out_OUT_DEMDiagnosticEventManager.FreezeFrame5 : KIBES_Signal/KIBES_Signal  MBDS_LibraryBlock=on  DatabaseKey=2256  SignalName=OUT_DEMDiagnosticEventManager.FreezeFrame5  SymbolName=OUT_DEMDiagnosticEventManager_FreezeFrame5_002256  DataType=uint16  Init=0  Slope=1  Bias=0  DataSize=1  fpDataType=uint16  BlockIOType=Outport  DeviceType=0
  out_OUT_DEMDiagnosticEventManager.FreezeFrame6 : KIBES_Signal/KIBES_Signal  MBDS_LibraryBlock=on  DatabaseKey=2266  SignalName=OUT_DEMDiagnosticEventManager.FreezeFrame6  SymbolName=OUT_DEMDiagnosticEventManager_FreezeFrame6_002266  DataType=uint16  Init=0  Slope=1  Bias=0  DataSize=1  fpDataType=uint16  BlockIOType=Outport  DeviceType=0
  out_OUT_DEMDiagnosticEventManager.FreezeFrame7 : KIBES_Signal/KIBES_Signal  MBDS_LibraryBlock=on  DatabaseKey=2267  SignalName=OUT_DEMDiagnosticEventManager.FreezeFrame7  SymbolName=OUT_DEMDiagnosticEventManager_FreezeFrame7_002267  DataType=uint16  Init=0  Slope=1  Bias=0  DataSize=1  fpDataType=uint16  BlockIOType=Outport  DeviceType=0
  out_OUT_DEMDiagnosticEventManager.FreezeFrame8 : KIBES_Signal/KIBES_Signal  MBDS_LibraryBlock=on  DatabaseKey=2268  SignalName=OUT_DEMDiagnosticEventManager.FreezeFrame8  SymbolName=OUT_DEMDiagnosticEventManager_FreezeFrame8_002268  DataType=uint16  Init=0  Slope=1  Bias=0  DataSize=1  fpDataType=uint16  BlockIOType=Outport  DeviceType=0
  out_OUT_DEMDiagnosticEventManager.FreezeFrame9 : KIBES_Signal/KIBES_Signal  MBDS_LibraryBlock=on  DatabaseKey=2269  SignalName=OUT_DEMDiagnosticEventManager.FreezeFrame9  SymbolName=OUT_DEMDiagnosticEventManager_FreezeFrame9_002269  DataType=uint16  Init=0  Slope=1  Bias=0  DataSize=1  fpDataType=uint16  BlockIOType=Outport  DeviceType=0
  out_OUT_DEMDiagnosticEventManager.OperationCycle : KIBES_Signal/KIBES_Signal  MBDS_LibraryBlock=on  DatabaseKey=2235  SignalName=OUT_DEMDiagnosticEventManager.OperationCycle  SymbolName=OUT_DEMDiagnosticEventManager_OperationCycle_002235  DataType=boolean  Init=0  Slope=1  Bias=0  DataSize=1  fpDataType=boolean  BlockIOType=Outport  DeviceType=0
  out_OUT_DEMDiagnosticEventManager.StorageCondition00 : KIBES_Signal/KIBES_Signal  MBDS_LibraryBlock=on  DatabaseKey=2240  SignalName=OUT_DEMDiagnosticEventManager.StorageCondition00  SymbolName=OUT_DEMDiagnosticEventManager_StorageCondition00_002240  DataType=boolean  Init=0  Slope=1  Bias=0  DataSize=1  fpDataType=boolean  BlockIOType=Outport  DeviceType=0
  out_OUT_DEMDiagnosticEventManager.StorageCondition01 : KIBES_Signal/KIBES_Signal  MBDS_LibraryBlock=on  DatabaseKey=2258  SignalName=OUT_DEMDiagnosticEventManager.StorageCondition01  SymbolName=OUT_DEMDiagnosticEventManager_StorageCondition01_002258  DataType=boolean  Init=0  Slope=1  Bias=0  DataSize=1  fpDataType=boolean  BlockIOType=Outport  DeviceType=0
  out_OUT_DEMDiagnosticEventManager.StorageCondition02 : KIBES_Signal/KIBES_Signal  MBDS_LibraryBlock=on  DatabaseKey=2259  SignalName=OUT_DEMDiagnosticEventManager.StorageCondition02  SymbolName=OUT_DEMDiagnosticEventManager_StorageCondition02_002259  DataType=boolean  Init=0  Slope=1  Bias=0  DataSize=1  fpDataType=boolean  BlockIOType=Outport  DeviceType=0
  out_OUT_DEMDiagnosticEventManager.StorageCondition03 : KIBES_Signal/KIBES_Signal  MBDS_LibraryBlock=on  DatabaseKey=2260  SignalName=OUT_DEMDiagnosticEventManager.StorageCondition03  SymbolName=OUT_DEMDiagnosticEventManager_StorageCondition03_002260  DataType=boolean  Init=0  Slope=1  Bias=0  DataSize=1  fpDataType=boolean  BlockIOType=Outport  DeviceType=0
  out_OUT_DEMDiagnosticEventManager.StorageCondition04 : KIBES_Signal/KIBES_Signal  MBDS_LibraryBlock=on  DatabaseKey=2261  SignalName=OUT_DEMDiagnosticEventManager.StorageCondition04  SymbolName=OUT_DEMDiagnosticEventManager_StorageCondition04_002261  DataType=boolean  Init=0  Slope=1  Bias=0  DataSize=1  fpDataType=boolean  BlockIOType=Outport  DeviceType=0
  out_OUT_DEMDiagnosticEventManager.StorageCondition05 : KIBES_Signal/KIBES_Signal  MBDS_LibraryBlock=on  DatabaseKey=2262  SignalName=OUT_DEMDiagnosticEventManager.StorageCondition05  SymbolName=OUT_DEMDiagnosticEventManager_StorageCondition05_002262  DataType=boolean  Init=0  Slope=1  Bias=0  DataSize=1  fpDataType=boolean  BlockIOType=Outport  DeviceType=0
  out_OUT_DEMDiagnosticEventManager.StorageCondition06 : KIBES_Signal/KIBES_Signal  MBDS_LibraryBlock=on  DatabaseKey=2263  SignalName=OUT_DEMDiagnosticEventManager.StorageCondition06  SymbolName=OUT_DEMDiagnosticEventManager_StorageCondition06_002263  DataType=boolean  Init=0  Slope=1  Bias=0  DataSize=1  fpDataType=boolean  BlockIOType=Outport  DeviceType=0
  out_OUT_DEMDiagnosticEventManager.StorageCondition07 : KIBES_Signal/KIBES_Signal  MBDS_LibraryBlock=on  DatabaseKey=2264  SignalName=OUT_DEMDiagnosticEventManager.StorageCondition07  SymbolName=OUT_DEMDiagnosticEventManager_StorageCondition07_002264  DataType=boolean  Init=0  Slope=1  Bias=0  DataSize=1  fpDataType=boolean  BlockIOType=Outport  DeviceType=0
  out_OUT_DEMDiagnosticEventManager.StorageCondition08 : KIBES_Signal/KIBES_Signal  MBDS_LibraryBlock=on  DatabaseKey=2265  SignalName=OUT_DEMDiagnosticEventManager.StorageCondition08  SymbolName=OUT_DEMDiagnosticEventManager_StorageCondition08_002265  DataType=boolean  Init=0  Slope=1  Bias=0  DataSize=1  fpDataType=boolean  BlockIOType=Outport  DeviceType=0
  out_OUT_DEMDiagnosticEventManager.StorageCondition09 : KIBES_Signal/KIBES_Signal  MBDS_LibraryBlock=on  DatabaseKey=2257  SignalName=OUT_DEMDiagnosticEventManager.StorageCondition09  SymbolName=OUT_DEMDiagnosticEventManager_StorageCondition09_002257  DataType=boolean  Init=0  Slope=1  Bias=0  DataSize=1  fpDataType=boolean  BlockIOType=Outport  DeviceType=0
  out_OUT_PCAN.DM1_10.MessageEnable : KIBES_Signal/KIBES_Signal  MBDS_LibraryBlock=on  DatabaseKey=2229  SignalName=OUT_PCAN.DM1_10.MessageEnable  SymbolName=OUT_PCAN_DM1_10_MessageEnable_002229  DataType=boolean  Init=0  Slope=1  Bias=0  DataSize=1  fpDataType=boolean  BlockIOType=Outport  DeviceType=0
  out_OUT_PCAN.GenericDM1TxMessage.DeviceEnable : KIBES_Signal/KIBES_Signal  MBDS_LibraryBlock=on  DatabaseKey=2236  SignalName=OUT_PCAN.GenericDM1TxMessage.DeviceEnable  SymbolName=OUT_PCAN_GenericDM1TxMessage_DeviceEnable_002236  DataType=boolean  Init=0  Slope=1  Bias=0  DataSize=1  fpDataType=boolean  BlockIOType=Outport  DeviceType=0
  bo_Out : Outport  OutDataTypeStr=boolean
  wires:
  bo_In/1 -> Terminator/1
  Ground/1 -> bo_Out/1  "bo_Out"
  Constant/1 -> out_OUT_PCAN.DM1_10.MessageEnable/1
  in_IN_PCAN.DM1_10.MessageState/1 -> Terminator1/1
  in_IN_PCAN.DM1_10.ProtectLamp/1 -> Terminator2/1
  in_IN_PCAN.DM1_10.ProtectLampFlash/1 -> Terminator3/1
  in_IN_PCAN.DM1_10.MalfunctionIndicatorLamp/1 -> Terminator4/1
  in_IN_PCAN.DM1_10.MalfunctionIndicatorLampFlash/1 -> Terminator5/1
  in_IN_PCAN.DM1_10.AmberWarningLamp/1 -> Terminator6/1
  in_IN_PCAN.DM1_10.AmberWarningLampFlash/1 -> Terminator7/1
  in_IN_PCAN.DM1_10.RedStopLamp/1 -> Terminator8/1
  in_IN_PCAN.DM1_10.RedStopLampFlash/1 -> Terminator9/1
  in_IN_DM1_10.Filter.boFilter1/1 -> [boDm1Filter1]
  Constant1/1 -> out_OUT_PCAN.GenericDM1TxMessage.DeviceEnable/1
  [boDm1Filter1] -> Data Type Conversion/1
  Data Type Conversion/1 -> out_OUT_DEMDiagnosticEventManager.DEMList.DTC_01/1
  in_IN_DEMDiagnosticEventManager.DeviceState/1 -> Terminator10/1
  Constant2/1 -> out_OUT_DEMDiagnosticEventManager.FreezeFrame10/1, out_OUT_DEMDiagnosticEventManager.FreezeFrame9/1, out_OUT_DEMDiagnosticEventManager.FreezeFrame8/1, out_OUT_DEMDiagnosticEventManager.FreezeFrame7/1, out_OUT_DEMDiagnosticEventManager.FreezeFrame6/1, out_OUT_DEMDiagnosticEventManager.FreezeFrame5/1, out_OUT_DEMDiagnosticEventManager.FreezeFrame4/1, out_OUT_DEMDiagnosticEventManager.FreezeFrame3/1, out_OUT_DEMDiagnosticEventManager.FreezeFrame2/1, out_OUT_DEMDiagnosticEventManager.FreezeFrame1/1
  Constant3/1 -> out_OUT_DEMDiagnosticEventManager.DateAndTime/1, out_OUT_DEMDiagnosticEventManager.Distance/1
  Constant4/1 -> out_OUT_DEMDiagnosticEventManager.OperationCycle/1
  Constant5/1 -> out_OUT_DEMDiagnosticEventManager.EnableCondition09/1, out_OUT_DEMDiagnosticEventManager.EnableCondition08/1, out_OUT_DEMDiagnosticEventManager.EnableCondition07/1, out_OUT_DEMDiagnosticEventManager.EnableCondition06/1, out_OUT_DEMDiagnosticEventManager.EnableCondition05/1, out_OUT_DEMDiagnosticEventManager.EnableCondition04/1, out_OUT_DEMDiagnosticEventManager.EnableCondition03/1, out_OUT_DEMDiagnosticEventManager.EnableCondition02/1, out_OUT_DEMDiagnosticEventManager.EnableCondition01/1, out_OUT_DEMDiagnosticEventManager.EnableCondition00/1
  Constant6/1 -> out_OUT_DEMDiagnosticEventManager.StorageCondition09/1, out_OUT_DEMDiagnosticEventManager.StorageCondition08/1, out_OUT_DEMDiagnosticEventManager.StorageCondition07/1, out_OUT_DEMDiagnosticEventManager.StorageCondition06/1, out_OUT_DEMDiagnosticEventManager.StorageCondition05/1, out_OUT_DEMDiagnosticEventManager.StorageCondition04/1, out_OUT_DEMDiagnosticEventManager.StorageCondition03/1, out_OUT_DEMDiagnosticEventManager.StorageCondition02/1, out_OUT_DEMDiagnosticEventManager.StorageCondition01/1, out_OUT_DEMDiagnosticEventManager.StorageCondition00/1
